simulink model "tentativa_com_motor_DC"  (R2012b)
settings: Solver=ode45  StartTime=0.0  StopTime=3  RelTol=1e-3
libraries: BLDC x3
settings Model: Creator=h3now  LastModifiedBy=h3now

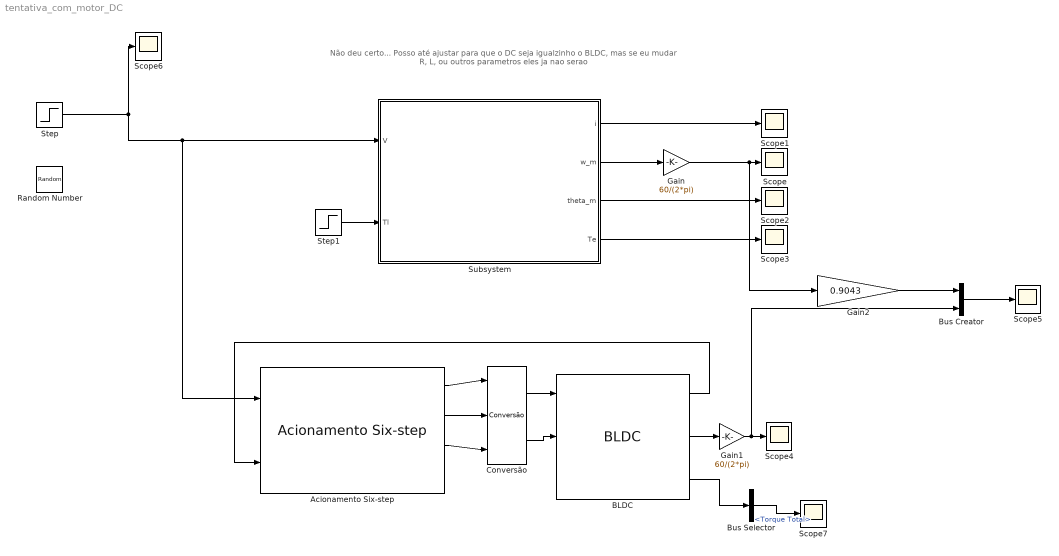
== system tentativa_com_motor_DC ==
  note: Não deu certo... Posso até ajustar para que o DC seja igualzinho o BLDC, mas se eu mudar R, L, ou outros parametros eles ja nao serao
  Acionamento Six-step : BLDC/Acionamento Six-step  P=8
  BLDC : BLDC/BLDC  J=3.84e-7  R=23.9/sqrt(3)  L=2.35e-3/sqrt(3)  P=8  Kt=11.3e-3  Ke=11.3e-3  Kd=0  default_fcem=on  fcem_a=fcem_a  fcem_b=fcem_b  fcem_c=fcem_c
  Bus Creator : BusCreator  Inputs=2
  Bus Selector : BusSelector  OutputSignals=Torque Total
  Conversão : BLDC/Conversão
  Gain : Gain  Gain=60/(2*pi)
  Gain1 : Gain  Gain=60/(2*pi)
  Gain2 : Gain  Gain=0.9043
  Random Number : RandomNumber  Variance=60  SampleTime=0.1
  Scope{,1..7} (8 alike) : Scope
      Scope2 settings: SaveName=ScopeData2
      Scope3 settings: SaveName=ScopeData3
      Scope4 settings: SaveName=ScopeData4
      Scope5 settings: TimeRange=3  YMin=-3000  YMax=4000  SaveName=ScopeData5
      Scope6 settings: SaveName=ScopeData6
      Scope7 settings: SaveName=ScopeData7
  Step : Step  Time=0  After=12  SampleTime=0
  Step1 : Step  Time=0  After=0  SampleTime=0
  Subsystem : Subsystem  mask{R=23.9, L=2.35e-3, J=3.84e-7, Kt=11.3e-3*0.9, Ke=11.3e-3, Kf=0}
      mask prompts: R "Resistência de armadura [Ohm]"; L "Indutância de armadura [H]"; J "Inércia do rotor [Kg/m^2]"; Kt "Constante de torque [N.m/A]"; Ke "Constante da força eletromotriz"; Kf "Constante de atrito viscoso"
      mask init:
      | A = [-R/L -Ke/L 0 ; Kt/J -Kf/J 0 ; 0 1 0];
      | B = [1/L 0 ; 0 -1/J ; 0 0];
      | C = [1 0 0 ; 0 1 0 ; 0 0 1 ; Kt 0 0];
      | D = zeros(4,2);
  wires:
  Step1/1 -> Subsystem/2(Tl)
  Subsystem/2(w_m) -> Gain/1
  Subsystem/1(i) -> Scope1/1
  Subsystem/3(theta_m) -> Scope2/1
  Subsystem/4(Te) -> Scope3/1
  Acionamento Six-step/1 -> Conversão/1
  Acionamento Six-step/2 -> Conversão/2
  Acionamento Six-step/3 -> Conversão/3
  Conversão/2 -> BLDC/2
  Conversão/1 -> BLDC/1
  BLDC/2 -> Gain1/1
  Gain1/1 -> Bus Creator/2, Scope4/1
  BLDC/1 -> Acionamento Six-step/2
  Bus Creator/1 -> Scope5/1
  Gain/1 -> Gain2/1, Scope/1
  Step/1 -> Acionamento Six-step/1, Subsystem/1(V), Scope6/1
  Gain2/1 -> Bus Creator/1
  BLDC/3 -> Bus Selector/1
  Bus Selector/1 -> Scope7/1  "<Torque Total>"

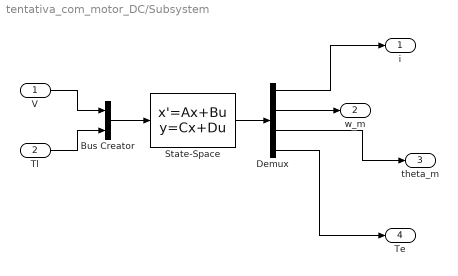
== system tentativa_com_motor_DC/Subsystem ==
  V : Inport
  Tl : Inport  Port=2
  Bus Creator : BusCreator  Inputs=2
  Demux : Demux
  State-Space : StateSpace  A=A  B=B  C=C  D=D
  i : Outport
  w_m : Outport  Port=2
  theta_m : Outport  Port=3
  Te : Outport  Port=4
  wires:
  State-Space/1 -> Demux/1
  Tl/1 -> Bus Creator/2
  V/1 -> Bus Creator/1
  Bus Creator/1 -> State-Space/1
  Demux/1 -> i/1
  Demux/3 -> theta_m/1
  Demux/2 -> w_m/1
  Demux/4 -> Te/1
